simulink model "networked"  (R2012a)
settings: Solver=ode45  StartTime=0.0  StopTime=2.0  RelTol=1e-3
libraries: truetime x4
settings Model: Creator=anton  LastModifiedBy=anton
settings DataIOCC: LimitDataPoints=on  SaveFormat=Array  ReturnWorkspaceOutputs=off
settings OptimizationCC: ExpressionDepthLimit=2147483647  LifeSpan=inf  SimCompilerOptimization=Off
settings DebuggingCC: UnderspecifiedInitializationDetection=Classic  MergeDetectMultiDrivingBlocksExec=none  SolverPrmCheckMsg=warning  FcnCallInpInsideContextMsg=Enable All  StateNameClashWarn=warning  SFUnexpectedBacktrackingDiag=warning  SFNoUnconditionalDefaultTransitionDiag=warning
settings HardwareCC: ProdBitPerPointer=32  ProdLargestAtomicFloat=None  ProdIntDivRoundTo=Undefined  ProdEndianess=Unspecified  ProdWordSize=32  ProdHWDeviceType=32-bit Generic
settings ModelReferenceCC: PropagateSignalLabelsOutOfModel=off
settings SFSimCC: SimUseLocalCustomCode=off
settings RTWCC: RTWUseLocalCustomCode=off  RTWCompilerOptimization=Off
settings GRTTargetCC: CodeReplacementLibrary=C89/C90 (ANSI)  GeneratePreprocessorConditionals=Disable all  CPPClassGenCompliant=off

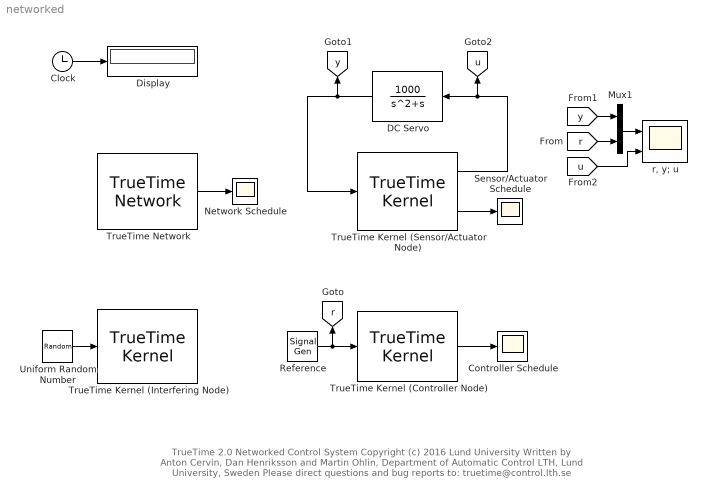
== system networked ==
  note: TrueTime 2.0  Networked Control System
      | Copyright (c) 2016 Lund University
      | Written by Anton Cervin, Dan Henriksson and Martin Ohlin,
      | Department of Automatic Control LTH, Lund University, Sweden
      | Please direct questions and bug reports to:  truetime@control.lth.se
  Clock : Clock
  Controller Schedule : Scope
      settings: TimeRange=2  MaxDataPoints=5000  SaveToWorkspace=off  SaveName=nschedule  YMin=0.5  YMax=4  SampleTime=-1
  DC Servo : TransferFcn  Numerator=[1000]  Denominator=[1 1 0]
  Display : Display
  Mux1 : Mux  Inputs=2
  Network Schedule : Scope
      settings: TimeRange=2  MaxDataPoints=5000  SaveToWorkspace=off  SaveName=nschedule1  YMin=1  YMax=3.5  SampleTime=-1
  Reference : SignalGenerator  WaveForm=square
  Sensor/Actuator Schedule : Scope
      settings: TimeRange=2  MaxDataPoints=5000  SaveToWorkspace=off  SaveName=nschedule2  YMin=0.5  YMax=4  SampleTime=-1
  TrueTime Kernel (Controller Node) : truetime/TrueTime Kernel  sfun=controller_init  args=0.0  ninputsoutputs=[1 0]  ntriggers=0  trigtype=rising  nwnodenbr=3  clockoffsetdrift=[0 0]  schedoutput=on  battery=off  poweroutput=off  label=1: 3
  TrueTime Kernel (Interfering Node) : truetime/TrueTime Kernel  sfun=interference_init  args=0.3  ninputsoutputs=[1 0]  ntriggers=0  trigtype=rising  nwnodenbr=1  clockoffsetdrift=[0 0]  schedoutput=off  battery=off  poweroutput=off  label=1: 1
  TrueTime Kernel (Sensor/Actuator Node) : truetime/TrueTime Kernel  sfun=sensor_actuator_init  args=[]  ninputsoutputs=[1 1]  ntriggers=0  trigtype=rising  nwnodenbr=2  clockoffsetdrift=[0 0]  schedoutput=on  battery=off  poweroutput=off  label=1: 2
  TrueTime Network : truetime/TrueTime Network  nwtype=CSMA/CD (Ethernet)  nwnbr=1  nnodes=3  rate=80000  minsize=80  lossprob=0  seed=0  bandwidths=[0.5 0.25 0.25]  slotsize=80  schedule=[1 2 1 3]  memsize=80000  buftype=Common buffer  overflow=Retransmit  dynSchedule=[]  miniSlotSize=40  NIT=0  QSortMode=FIFO  sync=0  irtSchedule=0  nrtLength=0  nodeGraph=0  scheduleoutput=on
  Uniform Random Number : UniformRandomNumber  Minimum=0  SampleTime=0.001
  "r, y; u" : Scope  NumInputPorts=2
      settings: TimeRange=2  MaxDataPoints=5000  SaveToWorkspace=off  SaveName=y  YMin=-2~-3  YMax=2~3  SampleTime=-1
  tag scope: r=global, u=global, y=global
  wires:
  TrueTime Network/1 -> Network Schedule/1
  Mux1/1 -> "r, y; u"/1
  Clock/1 -> Display/1
  Reference/1 -> TrueTime Kernel (Controller Node)/1, [r]
  TrueTime Kernel (Controller Node)/1 -> Controller Schedule/1
  [r] -> Mux1/2
  [y] -> Mux1/1
  [u] -> "r, y; u"/2
  Uniform Random Number/1 -> TrueTime Kernel (Interfering Node)/1
  TrueTime Kernel (Sensor/Actuator Node)/2 -> Sensor/Actuator Schedule/1
  DC Servo/1 -> TrueTime Kernel (Sensor/Actuator Node)/1, [y]
  TrueTime Kernel (Sensor/Actuator Node)/1 -> DC Servo/1, [u]
